simulink model "OnlineEDCPHILmodel"  (R2023a)
settings: Solver=ode8  StartTime=0.0  StopTime=100  FixedStep=1e-5  RelTol=1e-3
values from neighbouring files (symbols this model uses):
  CV = 1/(2*RV*xi*wn)    [OnlineEDCPHIL.m]
  ki = wn^2*RV*CV    [OnlineEDCPHIL.m]
  RV = 1    [OnlineEDCPHIL.m]
undefined symbols (not defined in the file or in its folder): Ion, Lithium
libraries: cstblocks x8, spsSeriesRLCBranchLib x7, spsCurrentMeasurementLib x5, spsIGBTDiodeLib x4, spsControlledCurrentSourceLib x2, spsFirstOrderFilterLib x2, spsGroundLib x2, spsPWMGeneratorDCDCLib x2, spsBatteryLib x1, spsControlledVoltageSourceLib x1, spsSupercapacitorLib x1, spsVoltageMeasurementLib x1
settings Model: Creator=USUARIO  LastModifiedBy=USUARIO

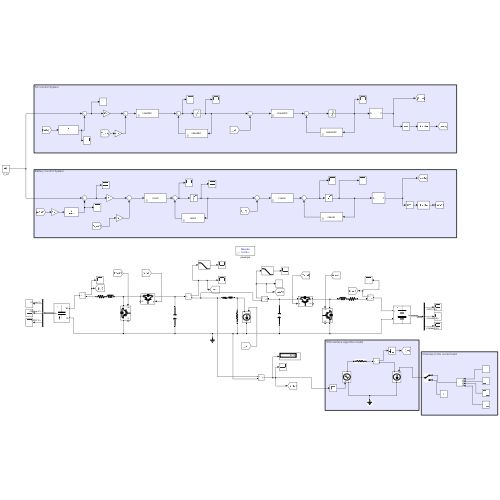
[thumbnail: Simulink's stored preview of the top-level diagram]
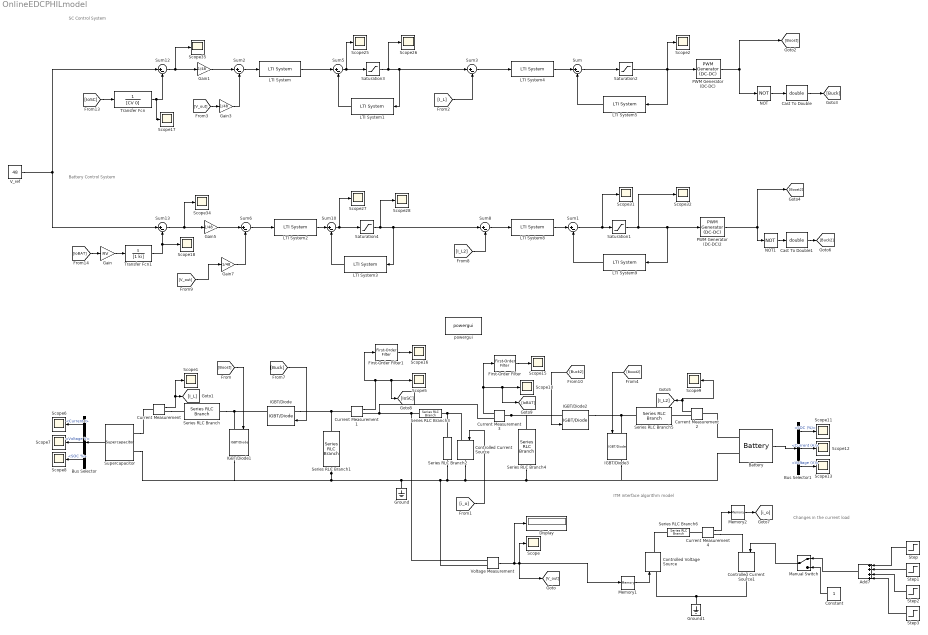
== system OnlineEDCPHILmodel ==
  note: Changes in the current load
  note: ITM interface algorithm model
  note: SC Control System
  note: Battery Control System
  Add7 : Sum  Inputs=++++
  Battery : spsBatteryLib/Battery  BatType=Lithium-Ion  ShowTempParam=off  ThermalPreset=no  ShowAgeParam=off  NomV=24  NomQ=15  SOC=40  Batt_Tr=30  PresetModel=on  MaxQ=15  MinV=18  FullV=27.9357  Dis_rate=6.5217  R=0.016  Normal_OP=13.5652  expZone="[25.9293     0.736957]"  current=[6.5 13 32.5]  Units=Time  Tci=20  NomT=20  T2=-30  MaxQ2=4.8  FullV2=7.1  Normal_OP2=5.655  expZone2="[6.58           1]"  Rca=0.6  ti=2000  Dp=0  Neq0=0  Tsim=1e6  Ta1=25  Qeol=5.4*0.9  Reol=0.013333*1.2  Char_age=[2.3478, 3]  Dis_age=[2.3478, 10]  N1=1500  N2=10500  N3=1000  N4=1400  Ta2=45  N5=950
  Bus Selector : BusSelector  OutputSignals=Current I,Voltage V,SOC %
  Bus Selector1 : BusSelector  OutputSignals=SOC (%),Current (A),Voltage (V)
  Cast To Double : DataTypeConversion  OutDataTypeStr=double  SaturateOnIntegerOverflow=off  RndMeth=Floor
  Cast To Double1 : DataTypeConversion  OutDataTypeStr=double  SaturateOnIntegerOverflow=off  RndMeth=Floor
  Constant : Constant
  Controlled Current Source : spsControlledCurrentSourceLib/Controlled Current Source  Initialize=on  Source_Type=DC  Amplitude=1  Phase=0  Frequency=0  Measurements=None
  Controlled Current Source1 : spsControlledCurrentSourceLib/Controlled Current Source  Initialize=on  Source_Type=DC  Amplitude=1  Phase=0  Frequency=0  Measurements=None
  Controlled Voltage Source : spsControlledVoltageSourceLib/Controlled Voltage Source  Initialize=off  Source_Type=DC  Amplitude=0  Phase=0  Frequency=0  Measurements=None
  Current Measurement{,1..4} (5 alike) : spsCurrentMeasurementLib/Current Measurement  PhasorSimulation=off  OutputType=Complex  PSBequivalent=0
  Display : Display
  First-Order Filter : spsFirstOrderFilterLib/First-Order Filter  FilterType=Lowpass  Tc=10e-2  Ts=0  Initialize=off  Vac_Init=[0, 0, 60]  Vdc_Init=0  PlotResponse=off  FreqRange="[0,  200,  1]"
  First-Order Filter1 : spsFirstOrderFilterLib/First-Order Filter  FilterType=Lowpass  Tc=10e-2  Ts=0  Initialize=off  Vac_Init=[0, 0, 60]  Vdc_Init=0  PlotResponse=off  FreqRange="[0,  200,  1]"
  Gain : Gain  Gain=RV
  Gain{1,3,5,7} (4 alike) : Gain  Gain=1/48
  Ground : spsGroundLib/Ground  LConnTagsString=a
  Ground1 : spsGroundLib/Ground  LConnTagsString=a
  IGBT/Diode{,1..3} (4 alike) : spsIGBTDiodeLib/IGBT//Diode  Ron=1e-3  Rs=1e6  Cs=inf  Measurements=on
  LTI System : cstblocks/LTI System  sys=c1antiSC  IC=[]
  LTI System1 : cstblocks/LTI System  sys=c2antiSC  IC=[]
  LTI System2 : cstblocks/LTI System  sys=c1anti  IC=[]
  LTI System3 : cstblocks/LTI System  sys=c2anti  IC=[]
  LTI System4 : cstblocks/LTI System  sys=c1anticSC  IC=[]
  LTI System5 : cstblocks/LTI System  sys=c2anticSC  IC=[]
  LTI System8 : cstblocks/LTI System  sys=c1antic  IC=[]
  LTI System9 : cstblocks/LTI System  sys=c2antic  IC=[]
  Manual Switch : ManualSwitch
  Memory1 : Memory
  Memory2 : Memory
  NOT : Logic  Operator=NOT  AllPortsSameDT=off  OutDataTypeStr=boolean
  NOT1 : Logic  Operator=NOT  AllPortsSameDT=off  OutDataTypeStr=boolean
  PWM Generator (DC-DC) : spsPWMGeneratorDCDCLib/PWM Generator (DC-DC)  Fsw=25000  Ts=0
  PWM Generator (DC-DC)2 : spsPWMGeneratorDCDCLib/PWM Generator (DC-DC)  Fsw=25000  Ts=0
  Saturation1 : Saturate  UpperLimit=0.95  LowerLimit=0.01
  Saturation2 : Saturate  UpperLimit=0.95  LowerLimit=0.01
  Saturation3 : Saturate  UpperLimit=10  LowerLimit=-10
  Saturation4 : Saturate  UpperLimit=12  LowerLimit=-12
  Scope{,1..2,5..13,15..18,25..28,31..32,34..35} (24 alike) : Scope
  Series RLC Branch : spsSeriesRLCBranchLib/Series RLC Branch  LConnTagsString=__new0  RConnTagsString=__new0  BranchType=RL  Resistance=1e-3  Inductance=8e-3  SetiL0=off  InitialCurrent=0  Capacitance=1e-6  Setx0=off  InitialVoltage=0  Measurements=None
  Series RLC Branch1 : spsSeriesRLCBranchLib/Series RLC Branch  LConnTagsString=__new0  RConnTagsString=__new0  BranchType=C  Resistance=1  Inductance=1e-3  SetiL0=off  InitialCurrent=0  Capacitance=0.0047  Setx0=off  InitialVoltage=0  Measurements=None
  Series RLC Branch2 : spsSeriesRLCBranchLib/Series RLC Branch  LConnTagsString=__new0  RConnTagsString=__new0  BranchType=R  Resistance=1e5  Inductance=1e-3  SetiL0=off  InitialCurrent=0  Capacitance=4700e-6  Setx0=off  InitialVoltage=0  Measurements=None
  Series RLC Branch3 : spsSeriesRLCBranchLib/Series RLC Branch  LConnTagsString=__new0  RConnTagsString=__new0  BranchType=RL  Resistance=1e-4  Inductance=75e-6  SetiL0=off  InitialCurrent=0  Capacitance=4700e-6  Setx0=off  InitialVoltage=0  Measurements=None
  Series RLC Branch4 : spsSeriesRLCBranchLib/Series RLC Branch  LConnTagsString=__new0  RConnTagsString=__new0  BranchType=C  Resistance=1  Inductance=1e-3  SetiL0=off  InitialCurrent=0  Capacitance=0.0047  Setx0=off  InitialVoltage=0  Measurements=None
  Series RLC Branch5 : spsSeriesRLCBranchLib/Series RLC Branch  LConnTagsString=__new0  RConnTagsString=__new0  BranchType=RL  Resistance=1e-3  Inductance=8e-3  SetiL0=off  InitialCurrent=0  Capacitance=1e-6  Setx0=off  InitialVoltage=0  Measurements=None
  Series RLC Branch6 : spsSeriesRLCBranchLib/Series RLC Branch  LConnTagsString=__new0  RConnTagsString=__new0  BranchType=R  Resistance=1e-3  Inductance=75e-6  SetiL0=off  InitialCurrent=0  Capacitance=4700e-6  Setx0=off  InitialVoltage=0  Measurements=None
  Step : Step  Time=0  SampleTime=0
  Step1 : Step  Time=37.82  After=2  SampleTime=0
  Step2 : Step  Time=69.7319  After=-2  SampleTime=0
  Step3 : Step  Time=95.9598  After=-2  SampleTime=0
  Sum{,1..3,5..6,8,10,12..13} (10 alike) : Sum  Inputs=|+-
  Supercapacitor : spsSupercapacitorLib/Supercapacitor  C=165  Rdc=6e-3  Voltage=48  Ns=18  Np=1  Vinit=24  Temp=25  PresetModel=off  EstParam=off  Nc=1  r=1e-9  epsilon=6.0208e-10  Ich=10  Vstern="[0.161  2.7  7.8]"  Self_dis=on  Ioc=10  Vself="[48  47.8  47.06  44.65]"  demandeplot=off  I="[10  20 100  500]"  Units=sec  Vmax=0  If=0  deltaV=0  alpha=0  sec=0
      settings: LibrarySourceBlock=sps_lib/Sources/Supercapacitor
  Transfer Fcn : TransferFcn  Denominator=[CV 0]
  Transfer Fcn1 : TransferFcn  Numerator=[1 0]  Denominator=[1 ki]
  V_ref : Constant  Value=48
  Voltage Measurement : spsVoltageMeasurementLib/Voltage Measurement  PhasorSimulation=off  OutputType=Complex  PSBequivalent=0
  powergui : spspowerguiLib/powergui  Priority=1  SimulationMode=Discrete  SampleTime=1e-5  frequency=60  Iterations=50  frequencyindice=0  Pbase=100e6  ErrMax=1e-4  UnitsV=kV  UnitsW=MW  buscounter=0  FunctionMessages=off  echomessages=off  EnableUseOfTLC=off  CurrentSourceSwitches=off  DisableSnubberDevices=off  DisableRonSwitches=off  DisableVfSwitches=off  DisplayEquations=off  AutomaticDiscreteSolvers=off  SolverType=Tustin/Backward Euler (TBE)  Interpol=off  ExternalGateDelay=off  methode=off  Ts=100  x0status=blocks  SPID=on  SwTol=0  HookPort=off  NonlinearTolerance=1e-4  nMaxIteration=100  ContinueOnMaxIteration=off  RestoreLinks=warning  ResistiveCurrentMeasurement=off  Frange=[0:2:500]  Ylog=off  Xlog=on  ShowGrid=off  save=off  variable=ZData  structure=0  ZoomFFT=off  StartTime=0.0  cycles=1  DisplayStyle=1  fundamental=60  FreqAxis=off  MaxFrequency=1000  frequencyindicesteady=1  RmsSteady=1  display=off
  wires:
  NOT/1 -> Cast To Double/1
  [Buck2] -> IGBT/Diode2/1
  Current Measurement1/1 -> [IoSC], Scope5/1, First-Order Filter1/1
  Current Measurement3/1 -> First-Order Filter/1, [IoBAT], Scope10/1
  [Boost] -> IGBT/Diode1/1
  Gain1/1 -> Sum2/1
  Step1/1 -> Add7/2
  LTI System2/1 -> Sum10/1
  [IoSC] -> Transfer Fcn/1
  Sum3/1 -> LTI System4/1
  Step2/1 -> Add7/3
  Step/1 -> Add7/1
  PWM Generator (DC-DC)2/1 -> [Boost2], NOT1/1
  Sum1/1 -> Saturation1/1, Scope31/1
  Step3/1 -> Add7/4
  Cast To Double/1 -> [Buck]
  Sum13/1 -> Scope34/1, Gain5/1
  NOT1/1 -> Cast To Double1/1
  PWM Generator (DC-DC)/1 -> [Boost], NOT/1
  Battery/1 -> Bus Selector1/1
  Sum2/1 -> LTI System/1
  [Boost2] -> IGBT/Diode3/1
  Transfer Fcn1/1 -> Scope18/1, Sum13/2
  LTI System9/1 -> Sum1/2
  Gain5/1 -> Sum6/1
  Saturation1/1 -> PWM Generator (DC-DC)2/1, LTI System9/1, Scope32/1
  Sum8/1 -> LTI System8/1
  Saturation3/1 -> Scope26/1, LTI System1/1, Sum3/1
  [IoBAT] -> Gain/1
  LTI System3/1 -> Sum10/2
  Sum12/1 -> Scope35/1, Gain1/1
  Voltage Measurement/1 -> Display/1, [V_out], Memory1/1, Scope/1
  Supercapacitor/1 -> Bus Selector/1
  Current Measurement/1 -> Scope1/1, [I_L]
  Bus Selector1/2 -> Scope12/1  "<Current (A)>"
  Saturation2/1 -> PWM Generator (DC-DC)/1, Scope2/1, LTI System5/1
  Transfer Fcn/1 -> Scope17/1, Sum12/2
  Cast To Double1/1 -> [Buck2]
  LTI System/1 -> Sum5/1
  Current Measurement2/1 -> Scope9/1, [I_L2]
  Sum6/1 -> LTI System2/1
  Bus Selector/2 -> Scope7/1  "<Voltage V>"
  LTI System8/1 -> Sum1/1
  V_ref/1 -> Sum13/1, Sum12/1
  LTI System4/1 -> Sum/1
  Bus Selector1/1 -> Scope11/1  "<SOC (%)>"
  Bus Selector/3 -> Scope8/1  "<SOC %>"
  Gain7/1 -> Sum6/2
  Sum/1 -> Saturation2/1
  Sum10/1 -> Saturation4/1, Scope27/1
  Gain3/1 -> Sum2/2
  Bus Selector1/3 -> Scope13/1  "<Voltage (V)>"
  LTI System1/1 -> Sum5/2
  Sum5/1 -> Saturation3/1, Scope25/1
  Saturation4/1 -> Scope28/1, Sum8/1, LTI System3/1
  [V_out] -> Gain3/1
  [Buck] -> IGBT/Diode/1
  Bus Selector/1 -> Scope6/1  "<Current I>"
  First-Order Filter1/1 -> Scope16/1
  LTI System5/1 -> Sum/2
  First-Order Filter/1 -> Scope15/1
  [I_L] -> Sum3/2
  [V_out] -> Gain7/1
  [I_L2] -> Sum8/2
  Gain/1 -> Transfer Fcn1/1
  Add7/1 -> Manual Switch/1
  Constant/1 -> Manual Switch/2
  Manual Switch/1 -> Controlled Current Source1/1
  Current Measurement4/1 -> Memory2/1
  [i_o] -> Controlled Current Source/1
  Memory1/1 -> Controlled Voltage Source/1
  Memory2/1 -> [i_o]
  connections:
  Series RLC Branch2/LConn1 -- Series RLC Branch3/RConn1 -- Controlled Current Source/LConn1
  Current Measurement3/LConn1 -- IGBT/Diode2/LConn1 -- Series RLC Branch4/LConn1
  Series RLC Branch1/RConn1 -- Supercapacitor/LConn2 -- IGBT/Diode1/RConn1 -- Controlled Current Source/RConn1 -- IGBT/Diode3/RConn1 -- Battery/LConn2 -- Series RLC Branch4/RConn1 -- Series RLC Branch2/RConn1 -- Voltage Measurement/LConn2 -- Ground/LConn1
  Current Measurement1/LConn1 -- IGBT/Diode/LConn1 -- Series RLC Branch1/LConn1
  IGBT/Diode2/RConn1 -- Series RLC Branch5/RConn1 -- IGBT/Diode3/LConn1
  Series RLC Branch/RConn1 -- IGBT/Diode1/LConn1 -- IGBT/Diode/RConn1
  Current Measurement2/RConn1 -- Series RLC Branch5/LConn1
  Voltage Measurement/LConn1 -- Current Measurement3/RConn1 -- Current Measurement1/RConn1 -- Series RLC Branch3/LConn1
  Current Measurement/RConn1 -- Series RLC Branch/LConn1
  Supercapacitor/LConn1 -- Current Measurement/LConn1
  Battery/LConn1 -- Current Measurement2/LConn1
  Controlled Voltage Source/RConn1 -- Series RLC Branch6/LConn1
  Controlled Current Source1/RConn1 -- Controlled Voltage Source/LConn1 -- Ground1/LConn1
  Current Measurement4/LConn1 -- Series RLC Branch6/RConn1
  Current Measurement4/RConn1 -- Controlled Current Source1/LConn1
